simulink model "IO_FBL_LQR"  (R2023b)
settings: Solver=VariableStepAuto  StartTime=0.0  StopTime=tf  RelTol=1e-6
values from neighbouring files (symbols this model uses):
  b = B/A    [ShipFinStabilizers.m]    (also in analisi_LUCIA.m = 1; plotRoutine.m = B/A*(1+uncertainty_perc))
  c = C/A    [ShipFinStabilizers.m]    (also in plotRoutine.m = C/A*(1+uncertainty_perc))
  controller_on = 0    [off.m]    (also in on.m = 1; plotRoutine.m)
  d = D/A    [ShipFinStabilizers.m]    (also in analisi_LUCIA.m = -0.1; plotRoutine.m = D/A*(1+uncertainty_perc))
  f = F/A    [ShipFinStabilizers.m]    (also in plotRoutine.m = F/A*(1+uncertainty_perc))
  Fw = 0.05    [ShipFinStabilizers.m]    (also in plotRoutine.m = 0.1)
  omega_w = 0.3    [ShipFinStabilizers.m]    (also in plotRoutine.m = 1.3)
  sat = 20    [ShipFinStabilizers.m]
  x0 = [deg2rad(10);0]    [ShipFinStabilizers.m]    (also in plotRoutine.m)
undefined symbols (not defined in the file or in its folder): A, B, C, D, F
settings Model: Creator=valen  LastModifiedBy=valen

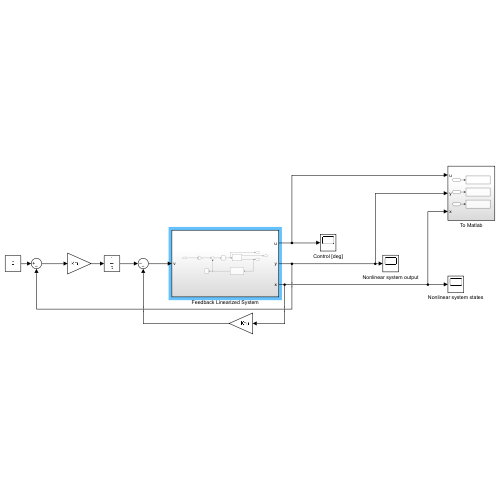
[thumbnail: Simulink's stored preview of the top-level diagram]
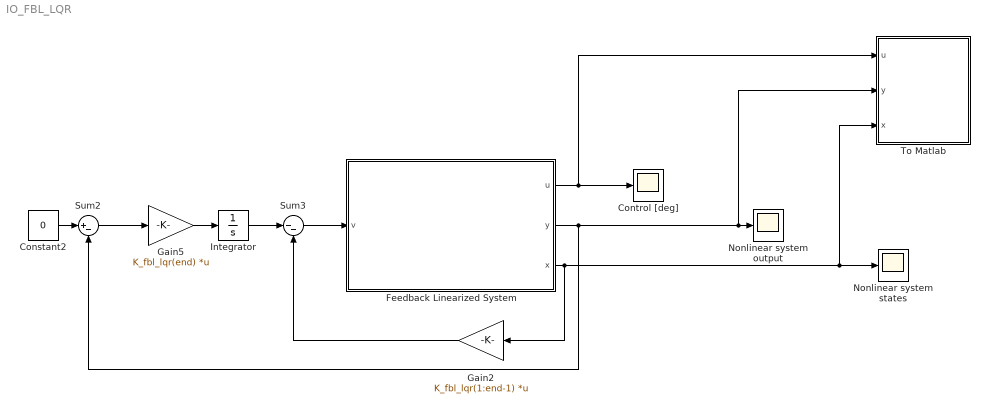
== system IO_FBL_LQR ==
  Constant2 : Constant  Value=0
  Control [deg] : Scope
  Feedback Linearized System : Subsystem
  Gain2 : Gain  Gain=K_fbl_lqr(1:end-1)  Multiplication=Matrix(K*u)
  Gain5 : Gain  Gain=K_fbl_lqr(end)  Multiplication=Matrix(K*u)
  Integrator : Integrator
  Nonlinear system output : Scope
  Nonlinear system states : Scope
  Sum2 : Sum  Inputs=|+-
  Sum3 : Sum  Inputs=|--
  To Matlab : Subsystem
  wires:
  Gain5/1 -> Integrator/1
  Gain2/1 -> Sum3/2
  Constant2/1 -> Sum2/1
  Integrator/1 -> Sum3/1
  Sum2/1 -> Gain5/1
  Feedback Linearized System/1(u) -> To Matlab/1(u), Control [deg]/1
  Feedback Linearized System/3(x) -> Gain2/1, To Matlab/3(x), Nonlinear system states/1
  Feedback Linearized System/2(y) -> Sum2/2, To Matlab/2(y), Nonlinear system output/1
  Sum3/1 -> Feedback Linearized System/1(v)

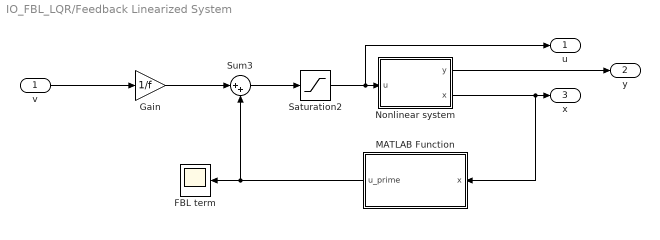
== system IO_FBL_LQR/Feedback Linearized System ==
  v : Inport
  FBL term : Scope
  Gain : Gain  Gain=1/f
  MATLAB Function : MATLAB Function  TreatAsAtomicUnit=on
  Nonlinear system : Subsystem
  Saturation2 : Saturate  UpperLimit=sat  LowerLimit=-sat
  Sum3 : Sum  Inputs=|++
  u : Outport
  y : Outport  Port=2
  x : Outport  Port=3
  wires:
  Nonlinear system/1(y) -> y/1
  MATLAB Function/1(u_prime) -> Sum3/2, FBL term/1
  Nonlinear system/2(x) -> x/1, MATLAB Function/1(x)
  Gain/1 -> Sum3/1
  Sum3/1 -> Saturation2/1
  Saturation2/1 -> u/1, Nonlinear system/1(u)
  v/1 -> Gain/1

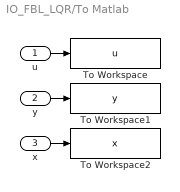
== system IO_FBL_LQR/To Matlab ==
  u : Inport  PortDimensions=1
  y : Inport  Port=2  PortDimensions=1
  x : Inport  Port=3  PortDimensions=[2,1]
  To Workspace : ToWorkspace  VariableName=u  SaveFormat=Structure With Time  SampleTime=-1
  To Workspace1 : ToWorkspace  VariableName=y  SaveFormat=Structure With Time  SampleTime=-1
  To Workspace2 : ToWorkspace  VariableName=x  SaveFormat=Structure With Time  SampleTime=-1
  wires:
  u/1 -> To Workspace/1
  x/1 -> To Workspace2/1
  y/1 -> To Workspace1/1

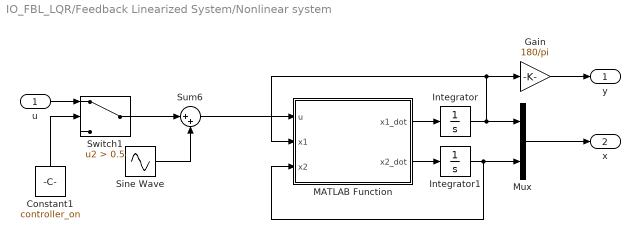
== system IO_FBL_LQR/Feedback Linearized System/Nonlinear system ==
  u : Inport
  Constant1 : Constant  Value=controller_on
  Gain : Gain  Gain=180/pi
  Integrator : Integrator  InitialCondition=x0(1)
  Integrator1 : Integrator  InitialCondition=x0(2)
  MATLAB Function : MATLAB Function  TreatAsAtomicUnit=on
  Mux : Mux  Inputs=2
  Sine Wave : Sin  Amplitude=Fw/F*A  Frequency=omega_w  SampleTime=0
  Sum6 : Sum  Inputs=|++
  Switch1 : Switch  Criteria=u2 > Threshold  Threshold=0.5  SaturateOnIntegerOverflow=off  InputSameDT=off
  y : Outport
  x : Outport  Port=2
  wires:
  Gain/1 -> y/1
  Mux/1 -> x/1
  MATLAB Function/1(x1_dot) -> Integrator/1
  MATLAB Function/2(x2_dot) -> Integrator1/1
  Integrator/1 -> MATLAB Function/2(x1), Gain/1, Mux/1
  Integrator1/1 -> MATLAB Function/3(x2), Mux/2
  Sum6/1 -> MATLAB Function/1(u)
  Switch1/1 -> Sum6/1
  u/1 -> Switch1/1
  Sine Wave/1 -> Sum6/2
  Constant1/1 -> Switch1/2

== matlab function IO_FBL_LQR/Feedback Linearized System/MATLAB Function ==
  data: x input size=[2;1]; u_prime output size=1; b parameter; c parameter; d parameter; e parameter; f parameter
function u_prime = fbl(x,b, c, d, e, f)

u_prime = 1/f*(-b*x(2) -c*x(2)*abs(x(2)) - d*x(1) - e*sin(x(1)));

== matlab function IO_FBL_LQR/Feedback Linearized System/Nonlinear system/MATLAB Function ==
  data: u input; x1_dot output; x1 input; x2 input; x2_dot output; A parameter; B parameter; C parameter; D parameter; E parameter; F parameter
function [x1_dot,x2_dot] = ship(u,x1,x2, A, B, C, D, E, F)

    x1_dot = x2;
    x2_dot = 1/A*( B*x2 + C*x2*abs(x2) + D*x1 + E*sin(x1) + F*u);
